simulink model "Laboratorio_1"  (R2024b)
settings: Solver=VariableStepAuto  StartTime=0.0  StopTime=10.0  RelTol=1e-3
settings Model: Creator=dayan  LastModifiedBy=dayan

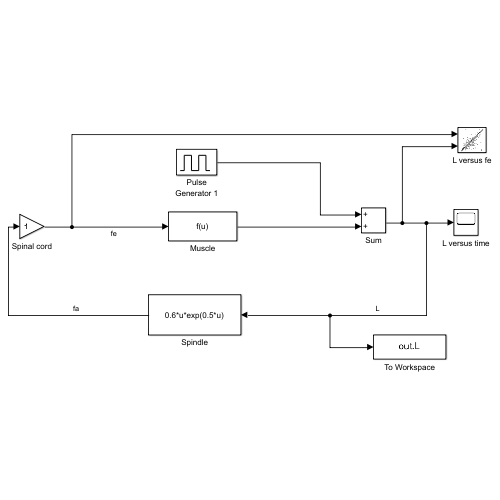
[thumbnail: Simulink's stored preview of the top-level diagram]
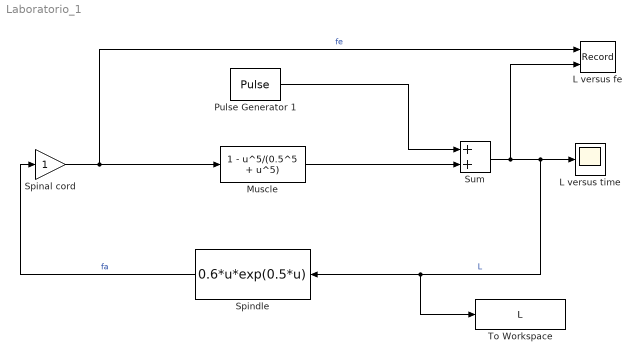
== system Laboratorio_1 ==
  L versus fe : Record  FileSettingsInternal="{\"entries\":[{\"content\":{\"excelSettings\":{\"content\":{},\"type\":\"Streamout.ExcelSettings\"}},\"type\":\"Streamout.FileSettingStorage\",\"uuid\":\"\"}],\"packageUris\":[\"http:\\/\\/schema.mathworks.com\\/mf0\\/streamout_blocks\\/R2020a\"],\"version\":\"1.0\"}"  Layout=[1 1]  SignalsInternal="{\"entries\":[{\"content\":{\"signals\":[{\"content\":{\"blockPath\":[],\"dimensions\":[1],\"domain\":\"\",\"lineColor\":\"#a2142f\",\"plots\":[ 1 ],\"port\":1,\"signalID\":1,\"signalName\":\"XY Graph:1\"},\"type\":\"RecordBlkView.Signal\",\"uuid\":\"\"},{\"content\":{\"blockPath\":[],\"dimensions\":[1],\"domain\":\"\",\"lineColor\":\"#139fff\",\"plots\":[ 1 ],\"port\":2,\"signalID\":2,\"signalName\":\"XY Graph:2\"},\"type\":\"RecordBlkView.Signal\",\"uuid\":\"\"}]},\"type\":\"RecordBlkView.InputSignals\",\"uuid\":\"\"}],\"packageUris\":[\"http:\\/\\/schema.mathworks.com\\/mf0\\/streamout_blocks\\/R2020a\"],\"version\":\"1.0\"}"  VisualizationBindings="{\"xyplotplugin\":{\"info\":[{\"series\":[{\"bindingParametersList\":[{\"parameter\":\"X-Axis\",\"signalID\":1,\"signalName\":\"XY Graph:1\"},{\"parameter\":\"Y-Axis\",\"signalID\":2,\"signalName\":\"XY Graph:2\"}],\"seriesID\":0}],\"subplotID\":1}]}}"  CompatibilityTag=XY
  L versus time : Scope
  Muscle : Fcn  Expr="1 -  u^5/(0.5^5  + u^5)"
  Pulse Generator 1 : DiscretePulseGenerator  PulseType=Time based  Period=15  PulseWidth=0.75
  Spinal cord : Gain
  Spindle : Fcn  Expr=0.6*u*exp(0.5*u)
  Sum : Sum
  To Workspace : ToWorkspace  VariableName=L  SampleTime=-1
  wires:
  Spinal cord/1 -> L versus fe/1, Muscle/1  "fe"
  Muscle/1 -> Sum/2
  Pulse Generator 1/1 -> Sum/1
  Sum/1 -> L versus fe/2, To Workspace/1, Spindle/1, L versus time/1  "L"
  Spindle/1 -> Spinal cord/1  "fa"
